simulink model "Plant_Model0"  (R2020a)
settings: Solver=ode45  StartTime=0.0  StopTime=120  RelTol=1e-3
values from neighbouring files (symbols this model uses):
  b = 50.0    [data.sldd]    (also in para3.m = 50)
  m = 1000.0    [data.sldd]    (also in para3.m = 1000)
settings Model: DataDictionary=data.sldd  Creator=vijay  LastModifiedBy=vijay
settings DataIOCC: SaveOutput=off  SaveTime=off

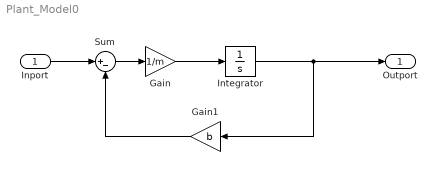
== system Plant_Model0 ==
  Inport : Inport  OutDataTypeStr=double  PortDimensions=1  SampleTime=0
  Gain : Gain  Gain=1/m
  Gain1 : Gain  Gain=b
  Integrator : Integrator
  Sum : Sum  Inputs=|+-
  Outport : Outport  OutDataTypeStr=double  PortDimensions=1  SampleTime=0
  wires:
  Sum/1 -> Gain/1
  Gain/1 -> Integrator/1
  Integrator/1 -> Gain1/1, Outport/1
  Gain1/1 -> Sum/2
  Inport/1 -> Sum/1
